simulink model "H2_Q3"  (R2019b)
settings: Solver=VariableStepAuto  StartTime=0.0  StopTime=10.0  RelTol=1e-3
values from neighbouring files (symbols this model uses):
  b = 100    [H2_Q1b.m]    (also in H2_Q1c.m = bandwidth(new); H2_Q1d1.m = bandwidth(new))
  m = 1000    [H2_Q1b.m]
settings Model: Creator=aravind  LastModifiedBy=aravind

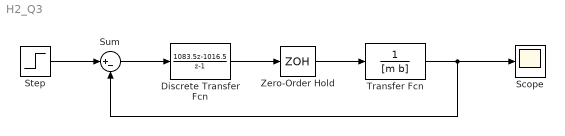
== system H2_Q3 ==
  Discrete Transfer Fcn : DiscreteTransferFcn  Numerator=[1083.5 -1016.5]  Denominator=[1 -1]
  Scope : Scope
  Step : Step  Time=0  SampleTime=0
  Sum : Sum  Inputs=|+-
  Transfer Fcn : TransferFcn  Denominator=[m b]
  Zero-Order Hold : ZeroOrderHold  SampleTime=0.1
  wires:
  Step/1 -> Sum/1
  Sum/1 -> Discrete Transfer Fcn/1
  Transfer Fcn/1 -> Sum/2, Scope/1
  Zero-Order Hold/1 -> Transfer Fcn/1
  Discrete Transfer Fcn/1 -> Zero-Order Hold/1
